simulink model "Task6"  (R2022a)
settings: Solver=VariableStepAuto  StartTime=0.0  StopTime=30  RelTol=1e-3
settings Model: Creator=Family  LastModifiedBy=Family

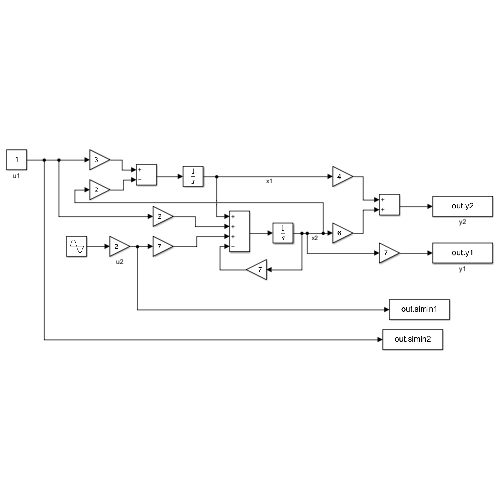
[thumbnail: Simulink's stored preview of the top-level diagram]
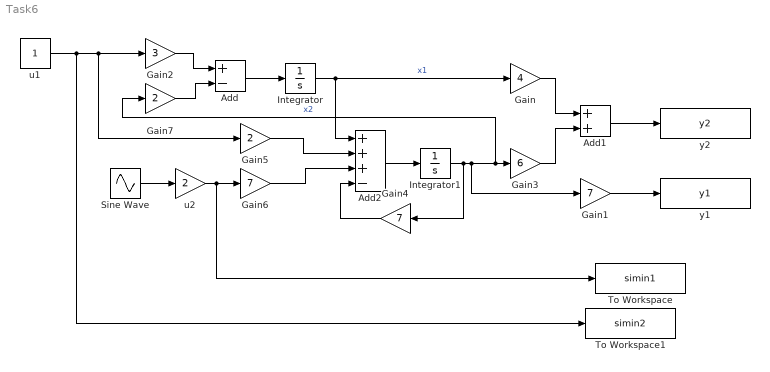
== system Task6 ==
  Add : Sum  Inputs=+-
  Add1 : Sum
  Add2 : Sum  Inputs=+++-
  Gain : Gain  Gain=4
  Gain1 : Gain  Gain=7
  Gain2 : Gain  Gain=3
  Gain3 : Gain  Gain=6
  Gain4 : Gain  Gain=7
  Gain5 : Gain  Gain=2
  Gain6 : Gain  Gain=7
  Gain7 : Gain  Gain=2
  Integrator : Integrator
  Integrator1 : Integrator
  Sine Wave : Sin  SampleTime=0
  To Workspace : ToWorkspace  VariableName=simin1  SaveFormat=Timeseries  SampleTime=-1
  To Workspace1 : ToWorkspace  VariableName=simin2  SaveFormat=Timeseries  SampleTime=-1
  u1 : Constant  SampleTime=-1
  u2 : Gain  Gain=2
  y1 : ToWorkspace  VariableName=y1  SaveFormat=Timeseries  SampleTime=-1
  y2 : ToWorkspace  VariableName=y2  SaveFormat=Timeseries  SampleTime=-1
  wires:
  Sine Wave/1 -> u2/1
  Gain1/1 -> y1/1
  Add/1 -> Integrator/1
  u1/1 -> To Workspace1/1, Gain5/1, Gain2/1
  Gain2/1 -> Add/1
  Add1/1 -> y2/1
  Gain/1 -> Add1/1
  Integrator/1 -> Add2/1, Gain/1  "x1"
  Integrator1/1 -> Gain7/1, Gain3/1, Gain1/1, Gain4/1  "x2"
  Gain3/1 -> Add1/2
  Add2/1 -> Integrator1/1
  Gain4/1 -> Add2/4
  Gain5/1 -> Add2/2
  Gain6/1 -> Add2/3
  u2/1 -> To Workspace/1, Gain6/1
  Gain7/1 -> Add/2
